simulink model "MpptInterferenceObservationMethod"  (R2024b)
settings: Solver=VariableStepAuto  StartTime=0.0  StopTime=3  RelTol=1e-3
libraries: spsSeriesRLCBranchLib x4, spsCurrentMeasurementLib x1, spsDiodeLib x1, spsMosfetLib x1, spsMultimeterLib x1, spsPVArrayLib x1, eePwmGenerator x1, simulink x1, spsVoltageMeasurementLib x1, sps_lib x1
settings Model: Creator=User  LastModifiedBy=User

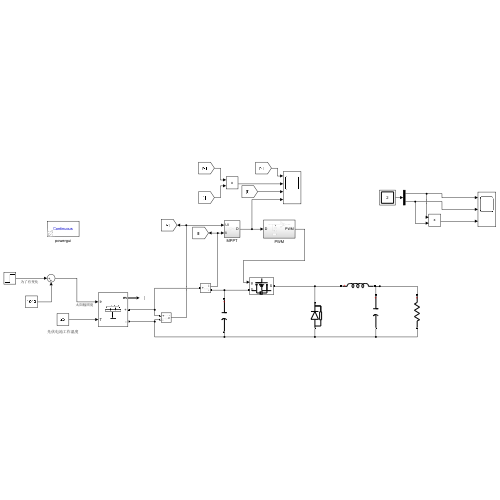
[thumbnail: Simulink's stored preview of the top-level diagram]
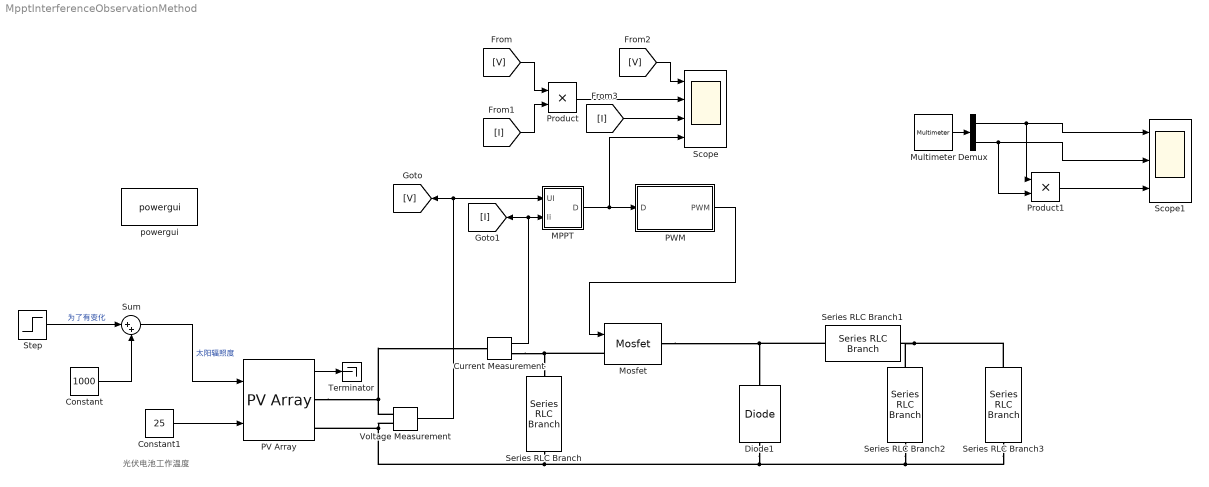
== system MpptInterferenceObservationMethod ==
  note: 光伏电池工作温度
  Constant : Constant  Value=1000
  Constant1 : Constant  Value=25
  Current Measurement : spsCurrentMeasurementLib/Current Measurement  PhasorSimulation=off  OutputType=Complex  PSBequivalent=0
  Demux : Demux  Outputs=2
  Diode1 : spsDiodeLib/Diode  Ron=0.001  Lon=0  Vf=0.8  IC=0  UseSnubber=0  Rs=500  Cs=250e-9  Measurements=off
  MPPT : Subsystem
  Mosfet : spsMosfetLib/Mosfet  Ron=0.1  Lon=0  Rd=0.01  Vfd=0  IC=0  Rs=1e5  Cs=inf  Measurements=off
  Multimeter : spsMultimeterLib/Multimeter  L=2  sel=[1 2]  yselected={}  Gain=[1 1]  OutputType=Complex  PlotAtSimulationStop=off  PhasorSimulation=off
  PV Array : spsPVArrayLib/PV Array  Npar=1  Nser=1  PlotType=array @ 25 deg.C & specified irradiances  S_vec="[ 1000  500  100 ]"  Temp_C_vec="[ 45 25  ]"  ModuleName=User-defined  PlotWhenSelected=off  Pm=213.15  Ncell=60  Voc=36.3  Isc=7.84  Vm=29  Im=7.35  beta_Voc_pc=-0.36099  alpha_Isc_pc=0.102  beta_Voc=-0.13104  alpha_Isc=0.0079968  IL=7.8654  I0=2.9273e-10  nI=0.98119  Rsh=313.0553  Rs=0.39381  RobustModel=off  RobustCellTemperature=313.3991  BAL=on  Tc=1e-6  Tfilter=5e-5
  PWM : Subsystem
  Product : Product
  Product1 : Product
  Scope : Scope  NumInputPorts=4
  Scope1 : Scope  NumInputPorts=3
  Series RLC Branch : spsSeriesRLCBranchLib/Series RLC Branch  LConnTagsString=__new0  RConnTagsString=__new0  BranchType=C  Resistance=1  Inductance=1e-3  SetiL0=off  InitialCurrent=0  Capacitance=1e-3  Setx0=off  InitialVoltage=0  Measurements=None
  Series RLC Branch1 : spsSeriesRLCBranchLib/Series RLC Branch  LConnTagsString=__new0  RConnTagsString=__new0  BranchType=L  Resistance=1  Inductance=1e-3  SetiL0=off  InitialCurrent=0  Capacitance=1e-6  Setx0=off  InitialVoltage=0  Measurements=None
  Series RLC Branch2 : spsSeriesRLCBranchLib/Series RLC Branch  LConnTagsString=__new0  RConnTagsString=__new0  BranchType=C  Resistance=1  Inductance=1e-3  SetiL0=off  InitialCurrent=0  Capacitance=1e-3  Setx0=off  InitialVoltage=0  Measurements=None
  Series RLC Branch3 : spsSeriesRLCBranchLib/Series RLC Branch  LConnTagsString=__new0  RConnTagsString=__new0  BranchType=R  Resistance=1  Inductance=1e-3  SetiL0=off  InitialCurrent=0  Capacitance=1e-6  Setx0=off  InitialVoltage=0  Measurements=Branch voltage and current
  Step : Step  Time=1.5  After=200  SampleTime=0
  Sum : Sum  Inputs=|++
  Terminator : Terminator
  Voltage Measurement : spsVoltageMeasurementLib/Voltage Measurement  PhasorSimulation=off  OutputType=Complex  PSBequivalent=0
  powergui : sps_lib/powergui  Priority=1  SimulationMode=Continuous  SampleTime=50e-6  frequency=60  Iterations=50  frequencyindice=0  Pbase=100e6  ErrMax=1e-4  UnitsV=kV  UnitsW=MW  buscounter=0  FunctionMessages=off  echomessages=off  EnableUseOfTLC=off  CurrentSourceSwitches=off  DisableSnubberDevices=off  DisableRonSwitches=off  DisableVfSwitches=off  DisplayEquations=off  AutomaticDiscreteSolvers=off  SolverType=Tustin/Backward Euler (TBE)  Interpol=off  ExternalGateDelay=off  methode=off  Ts=100  x0status=blocks  SPID=on  SwTol=0  HookPort=off  NonlinearTolerance=1e-4  nMaxIteration=100  ContinueOnMaxIteration=off  RestoreLinks=warning  ResistiveCurrentMeasurement=off  Frange=[0:2:500]  Ylog=off  Xlog=on  ShowGrid=off  save=off  variable=ZData  structure=0  ZoomFFT=off  StartTime=0.0  cycles=1  DisplayStyle=1  fundamental=60  FreqAxis=off  MaxFrequency=1000  frequencyindicesteady=1  RmsSteady=1  display=off
  wires:
  Constant1/1 -> PV Array/2
  PV Array/1 -> Terminator/1
  Step/1 -> Sum/1  "为了有变化"
  Constant/1 -> Sum/2
  Sum/1 -> PV Array/1  "太阳辐照度"
  Voltage Measurement/1 -> [V], MPPT/1(UI)
  Current Measurement/1 -> [I], MPPT/2(Ii)
  MPPT/1(D) -> Scope/4, PWM/1(D)
  [V] -> Product/1
  [I] -> Product/2
  Product/1 -> Scope/2
  [V] -> Scope/1
  [I] -> Scope/3
  PWM/1(PWM) -> Mosfet/1
  Multimeter/1 -> Demux/1
  Demux/1 -> Product1/1, Scope1/1
  Demux/2 -> Product1/2, Scope1/2
  Product1/1 -> Scope1/3
  connections:
  PV Array/RConn1 -- Voltage Measurement/LConn1 -- Current Measurement/LConn1
  Voltage Measurement/LConn2 -- Series RLC Branch3/RConn1 -- Series RLC Branch2/RConn1 -- Diode1/LConn1 -- Series RLC Branch/RConn1 -- PV Array/RConn2
  Current Measurement/RConn1 -- Mosfet/LConn1 -- Series RLC Branch/LConn1
  Mosfet/RConn1 -- Series RLC Branch1/LConn1 -- Diode1/RConn1
  Series RLC Branch2/LConn1 -- Series RLC Branch3/LConn1 -- Series RLC Branch1/RConn1

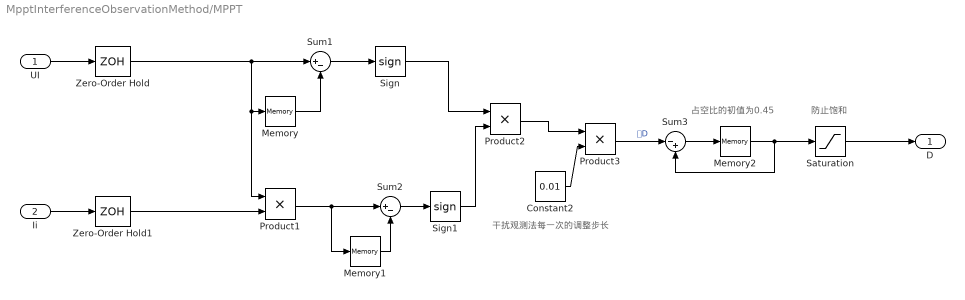
== system MpptInterferenceObservationMethod/MPPT ==
  note: 防止饱和
  note: 占空比的初值为0.45
  note: 干扰观测法每一次的调整步长
  UI : Inport
  Ii : Inport  Port=2
  Constant2 : Constant  Value=0.01
  Memory : Memory
  Memory1 : Memory
  Memory2 : Memory  InitialCondition=0.45
  Product1 : Product
  Product2 : Product
  Product3 : Product
  Saturation : Saturate  UpperLimit=1  LowerLimit=0
  Sign : Signum
  Sign1 : Signum
  Sum1 : Sum  Inputs=|+-
  Sum2 : Sum  Inputs=|+-
  Sum3 : Sum  Inputs=|-+
  Zero-Order Hold : ZeroOrderHold  SampleTime=0.05
  Zero-Order Hold1 : ZeroOrderHold  SampleTime=0.05
  D : Outport
  wires:
  Memory2/1 -> Saturation/1, Sum3/2
  Sum1/1 -> Sign/1
  Product3/1 -> Sum3/1  "🔺D"
  Zero-Order Hold/1 -> Product1/1, Memory/1, Sum1/1
  Sign/1 -> Product2/1
  Sum2/1 -> Sign1/1
  Product2/1 -> Product3/1
  Constant2/1 -> Product3/2
  Ii/1 -> Zero-Order Hold1/1
  Sum3/1 -> Memory2/1
  Sign1/1 -> Product2/2
  UI/1 -> Zero-Order Hold/1
  Product1/1 -> Memory1/1, Sum2/1
  Zero-Order Hold1/1 -> Product1/2
  Saturation/1 -> D/1
  Memory1/1 -> Sum2/2
  Memory/1 -> Sum1/2

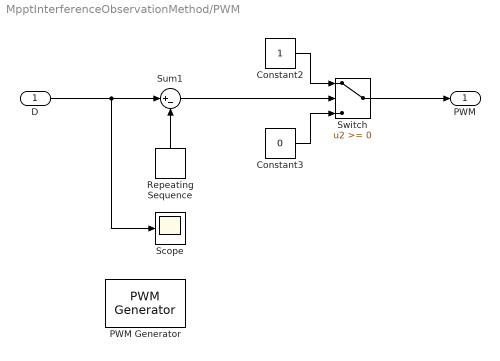
== system MpptInterferenceObservationMethod/PWM ==
  D : Inport
  Constant2 : Constant
  Constant3 : Constant  Value=0
  PWM Generator : eePwmGenerator/PWM Generator  CarrCount=Up  Tper=10000  Tdelay=0  Ts=5e-5
  Repeating Sequence : simulink/Sources/Repeating Sequence  rep_seq_t=[0 1e-4]  rep_seq_y=[0 1]
  Scope : Scope
  Sum1 : Sum  Inputs=|+-
  Switch : Switch  SaturateOnIntegerOverflow=off  InputSameDT=off
  PWM : Outport
  wires:
  Sum1/1 -> Switch/2
  D/1 -> Scope/1, Sum1/1
  Repeating Sequence/1 -> Sum1/2
  Constant3/1 -> Switch/3
  Constant2/1 -> Switch/1
  Switch/1 -> PWM/1
